simulink model "xieboduoji_13fangzhennow"  (R2023a)
settings: Solver=ode4  StartTime=0.0  StopTime=2.2  FixedStep=5e-7  RelTol=1e-3
undefined symbols (not defined in the file or in its folder): magnitude
libraries: simulink x417, spsRMSLib x70, spsCurrentMeasurementLib x32, spsVoltageMeasurementLib x31, powerlib_meascontrol x24, spsFourierLib x21, spsGroundLib x19, spsThreePhasePISectionLineLib x17, spsThreePhaseSeriesRLCBranchLib x14, spsdq0toAlphaBetaZeroLib x13, spsSeriesRLCBranchLib x11, spsUniversalBridgeLib x11
(part 10 of 12)

== system xieboduoji_13fangzhennow/node3/PV15kW2/谐波检测/DFT6-24A2/Sub5 ==
  In1 : Inport
  Constant{10,12,15,17} (4 alike) : Constant  Value=100*pi
  Constant11 : Constant  Value=19
  Cos : Trigonometry  Operator=cos
  Cos1 : Trigonometry  Operator=cos
  Cos2 : Trigonometry
  Cos3 : Trigonometry
  Delay : Delay  DelayLength=400  SampleTime=5e-5
  Delay1 : Delay  DelayLength=1  SampleTime=5e-5
  Delay2 : Delay  DelayLength=1  SampleTime=5e-5
  Divide{,1..3} (4 alike) : Product  Inputs=***
  Dot Product{,1..2,4} (4 alike) : DotProduct  OutDataTypeStr=Inherit: Inherit via internal rule
  Gain : Gain  Gain=2/400
  Gain10 : Gain  Gain=2/400
  Ramp{,1..3} (4 alike) : simulink/Sources/Ramp  slope=1  start=0  InitialOutput=0
  Sum18 : Sum  Inputs=|++
  Sum2 : Sum  Inputs=-+|
  Sum3 : Sum  Inputs=|++
  Sum9 : Sum  Inputs=|++
  Out1 : Outport
  wires:
  [thk] -> Divide/1
  Constant11/1 -> [thk]
  Sum9/1 -> Out1/1
  Dot Product1/1 -> Sum9/1
  Gain/1 -> Sum3/1
  Ramp2/1 -> Divide2/3
  Constant10/1 -> Divide/2
  Delay2/1 -> Sum18/2
  Gain10/1 -> Sum18/1
  Sum3/1 -> Delay1/1, Dot Product1/2
  Delay/1 -> Sum2/1
  Divide1/1 -> Cos1/1
  Ramp1/1 -> Divide1/3
  Constant12/1 -> Divide1/2
  Divide2/1 -> Cos2/1
  Cos3/1 -> Dot Product4/2
  Dot Product2/1 -> Gain10/1
  Cos2/1 -> Dot Product2/2
  Delay1/1 -> Sum3/2
  Divide3/1 -> Cos3/1
  Ramp3/1 -> Divide3/3
  [thk] -> Divide1/1
  Dot Product4/1 -> Sum9/2
  [thk] -> Divide2/1
  [thk] -> Divide3/1
  Sum18/1 -> Delay2/1, Dot Product4/1
  Constant15/1 -> Divide2/2
  In1/1 -> Sum2/2, Delay/1
  Cos1/1 -> Dot Product1/1
  Dot Product/1 -> Gain/1
  Cos/1 -> Dot Product/1
  Divide/1 -> Cos/1
  Sum2/1 -> Dot Product/2, Dot Product2/1
  Ramp/1 -> Divide/3
  Constant17/1 -> Divide3/2

== system xieboduoji_13fangzhennow/node3/PV15kW2/谐波检测/DFT6-24A3/Sub ==
  In1 : Inport
  Constant{10,12,15,17} (4 alike) : Constant  Value=100*pi
  Constant11 : Constant  Value=5
  Cos : Trigonometry  Operator=cos
  Cos1 : Trigonometry  Operator=cos
  Cos2 : Trigonometry
  Cos3 : Trigonometry
  Delay : Delay  DelayLength=400  SampleTime=5e-5
  Delay1 : Delay  DelayLength=1  SampleTime=5e-5
  Delay2 : Delay  DelayLength=1  SampleTime=5e-5
  Divide{,1..3} (4 alike) : Product  Inputs=***
  Dot Product{,1..2,4} (4 alike) : DotProduct  OutDataTypeStr=Inherit: Inherit via internal rule
  Gain : Gain  Gain=2/400
  Gain10 : Gain  Gain=2/400
  Ramp{,1..3} (4 alike) : simulink/Sources/Ramp  slope=1  start=0  InitialOutput=0
  Sum18 : Sum  Inputs=|++
  Sum2 : Sum  Inputs=-+|
  Sum3 : Sum  Inputs=|++
  Sum9 : Sum  Inputs=|++
  Out1 : Outport
  wires:
  Constant17/1 -> Divide3/2
  Ramp/1 -> Divide/3
  Sum2/1 -> Dot Product2/1, Dot Product/2
  Divide/1 -> Cos/1
  Cos/1 -> Dot Product/1
  Dot Product/1 -> Gain/1
  Cos1/1 -> Dot Product1/1
  In1/1 -> Delay/1, Sum2/2
  Constant15/1 -> Divide2/2
  Sum18/1 -> Dot Product4/1, Delay2/1
  [thk] -> Divide3/1
  [thk] -> Divide2/1
  Dot Product4/1 -> Sum9/2
  [thk] -> Divide1/1
  Ramp3/1 -> Divide3/3
  Divide3/1 -> Cos3/1
  Delay1/1 -> Sum3/2
  Cos2/1 -> Dot Product2/2
  Dot Product2/1 -> Gain10/1
  Cos3/1 -> Dot Product4/2
  Divide2/1 -> Cos2/1
  Constant12/1 -> Divide1/2
  Ramp1/1 -> Divide1/3
  Divide1/1 -> Cos1/1
  Delay/1 -> Sum2/1
  Sum3/1 -> Dot Product1/2, Delay1/1
  Gain10/1 -> Sum18/1
  Delay2/1 -> Sum18/2
  Constant10/1 -> Divide/2
  Ramp2/1 -> Divide2/3
  Gain/1 -> Sum3/1
  Dot Product1/1 -> Sum9/1
  Sum9/1 -> Out1/1
  Constant11/1 -> [thk]
  [thk] -> Divide/1

== system xieboduoji_13fangzhennow/node3/PV15kW2/谐波检测/DFT6-24A3/Sub1 ==
  In1 : Inport
  Constant{10,12,15,17} (4 alike) : Constant  Value=100*pi
  Constant11 : Constant  Value=7
  Cos : Trigonometry  Operator=cos
  Cos1 : Trigonometry  Operator=cos
  Cos2 : Trigonometry
  Cos3 : Trigonometry
  Delay : Delay  DelayLength=400  SampleTime=5e-5
  Delay1 : Delay  DelayLength=1  SampleTime=5e-5
  Delay2 : Delay  DelayLength=1  SampleTime=5e-5
  Divide{,1..3} (4 alike) : Product  Inputs=***
  Dot Product{,1..2,4} (4 alike) : DotProduct  OutDataTypeStr=Inherit: Inherit via internal rule
  Gain : Gain  Gain=2/400
  Gain10 : Gain  Gain=2/400
  Ramp{,1..3} (4 alike) : simulink/Sources/Ramp  slope=1  start=0  InitialOutput=0
  Sum18 : Sum  Inputs=|++
  Sum2 : Sum  Inputs=-+|
  Sum3 : Sum  Inputs=|++
  Sum9 : Sum  Inputs=|++
  Out1 : Outport
  wires:
  [thk] -> Divide/1
  Constant11/1 -> [thk]
  Sum9/1 -> Out1/1
  Dot Product1/1 -> Sum9/1
  Gain/1 -> Sum3/1
  Ramp2/1 -> Divide2/3
  Constant10/1 -> Divide/2
  Delay2/1 -> Sum18/2
  Gain10/1 -> Sum18/1
  Sum3/1 -> Delay1/1, Dot Product1/2
  Delay/1 -> Sum2/1
  Divide1/1 -> Cos1/1
  Ramp1/1 -> Divide1/3
  Constant12/1 -> Divide1/2
  Divide2/1 -> Cos2/1
  Cos3/1 -> Dot Product4/2
  Dot Product2/1 -> Gain10/1
  Cos2/1 -> Dot Product2/2
  Delay1/1 -> Sum3/2
  Divide3/1 -> Cos3/1
  Ramp3/1 -> Divide3/3
  [thk] -> Divide1/1
  Dot Product4/1 -> Sum9/2
  [thk] -> Divide2/1
  [thk] -> Divide3/1
  Sum18/1 -> Delay2/1, Dot Product4/1
  Constant15/1 -> Divide2/2
  In1/1 -> Sum2/2, Delay/1
  Cos1/1 -> Dot Product1/1
  Dot Product/1 -> Gain/1
  Cos/1 -> Dot Product/1
  Divide/1 -> Cos/1
  Sum2/1 -> Dot Product/2, Dot Product2/1
  Ramp/1 -> Divide/3
  Constant17/1 -> Divide3/2

== system xieboduoji_13fangzhennow/node3/PV15kW2/谐波检测/DFT6-24A3/Sub2 ==
  In1 : Inport
  Constant{10,12,15,17} (4 alike) : Constant  Value=100*pi
  Constant11 : Constant  Value=11
  Cos : Trigonometry  Operator=cos
  Cos1 : Trigonometry  Operator=cos
  Cos2 : Trigonometry
  Cos3 : Trigonometry
  Delay : Delay  DelayLength=400  SampleTime=5e-5
  Delay1 : Delay  DelayLength=1  SampleTime=5e-5
  Delay2 : Delay  DelayLength=1  SampleTime=5e-5
  Divide{,1..3} (4 alike) : Product  Inputs=***
  Dot Product{,1..2,4} (4 alike) : DotProduct  OutDataTypeStr=Inherit: Inherit via internal rule
  Gain : Gain  Gain=2/400
  Gain10 : Gain  Gain=2/400
  Ramp{,1..3} (4 alike) : simulink/Sources/Ramp  slope=1  start=0  InitialOutput=0
  Sum18 : Sum  Inputs=|++
  Sum2 : Sum  Inputs=-+|
  Sum3 : Sum  Inputs=|++
  Sum9 : Sum  Inputs=|++
  Out1 : Outport
  wires:
  Constant17/1 -> Divide3/2
  Ramp/1 -> Divide/3
  Sum2/1 -> Dot Product2/1, Dot Product/2
  Divide/1 -> Cos/1
  Cos/1 -> Dot Product/1
  Dot Product/1 -> Gain/1
  Cos1/1 -> Dot Product1/1
  In1/1 -> Delay/1, Sum2/2
  Constant15/1 -> Divide2/2
  Sum18/1 -> Dot Product4/1, Delay2/1
  [thk] -> Divide3/1
  [thk] -> Divide2/1
  Dot Product4/1 -> Sum9/2
  [thk] -> Divide1/1
  Ramp3/1 -> Divide3/3
  Divide3/1 -> Cos3/1
  Delay1/1 -> Sum3/2
  Cos2/1 -> Dot Product2/2
  Dot Product2/1 -> Gain10/1
  Cos3/1 -> Dot Product4/2
  Divide2/1 -> Cos2/1
  Constant12/1 -> Divide1/2
  Ramp1/1 -> Divide1/3
  Divide1/1 -> Cos1/1
  Delay/1 -> Sum2/1
  Sum3/1 -> Dot Product1/2, Delay1/1
  Gain10/1 -> Sum18/1
  Delay2/1 -> Sum18/2
  Constant10/1 -> Divide/2
  Ramp2/1 -> Divide2/3
  Gain/1 -> Sum3/1
  Dot Product1/1 -> Sum9/1
  Sum9/1 -> Out1/1
  Constant11/1 -> [thk]
  [thk] -> Divide/1

== system xieboduoji_13fangzhennow/node3/PV15kW2/谐波检测/DFT6-24A3/Sub3 ==
  In1 : Inport
  Constant{10,12,15,17} (4 alike) : Constant  Value=100*pi
  Constant11 : Constant  Value=13
  Cos : Trigonometry  Operator=cos
  Cos1 : Trigonometry  Operator=cos
  Cos2 : Trigonometry
  Cos3 : Trigonometry
  Delay : Delay  DelayLength=400  SampleTime=5e-5
  Delay1 : Delay  DelayLength=1  SampleTime=5e-5
  Delay2 : Delay  DelayLength=1  SampleTime=5e-5
  Divide{,1..3} (4 alike) : Product  Inputs=***
  Dot Product{,1..2,4} (4 alike) : DotProduct  OutDataTypeStr=Inherit: Inherit via internal rule
  Gain : Gain  Gain=2/400
  Gain10 : Gain  Gain=2/400
  Ramp{,1..3} (4 alike) : simulink/Sources/Ramp  slope=1  start=0  InitialOutput=0
  Sum18 : Sum  Inputs=|++
  Sum2 : Sum  Inputs=-+|
  Sum3 : Sum  Inputs=|++
  Sum9 : Sum  Inputs=|++
  Out1 : Outport
  wires:
  [thk] -> Divide/1
  Constant11/1 -> [thk]
  Sum9/1 -> Out1/1
  Dot Product1/1 -> Sum9/1
  Gain/1 -> Sum3/1
  Ramp2/1 -> Divide2/3
  Constant10/1 -> Divide/2
  Delay2/1 -> Sum18/2
  Gain10/1 -> Sum18/1
  Sum3/1 -> Delay1/1, Dot Product1/2
  Delay/1 -> Sum2/1
  Divide1/1 -> Cos1/1
  Ramp1/1 -> Divide1/3
  Constant12/1 -> Divide1/2
  Divide2/1 -> Cos2/1
  Cos3/1 -> Dot Product4/2
  Dot Product2/1 -> Gain10/1
  Cos2/1 -> Dot Product2/2
  Delay1/1 -> Sum3/2
  Divide3/1 -> Cos3/1
  Ramp3/1 -> Divide3/3
  [thk] -> Divide1/1
  Dot Product4/1 -> Sum9/2
  [thk] -> Divide2/1
  [thk] -> Divide3/1
  Sum18/1 -> Delay2/1, Dot Product4/1
  Constant15/1 -> Divide2/2
  In1/1 -> Sum2/2, Delay/1
  Cos1/1 -> Dot Product1/1
  Dot Product/1 -> Gain/1
  Cos/1 -> Dot Product/1
  Divide/1 -> Cos/1
  Sum2/1 -> Dot Product/2, Dot Product2/1
  Ramp/1 -> Divide/3
  Constant17/1 -> Divide3/2

== system xieboduoji_13fangzhennow/node3/PV15kW2/谐波检测/DFT6-24A3/Sub4 ==
  In1 : Inport
  Constant{10,12,15,17} (4 alike) : Constant  Value=100*pi
  Constant11 : Constant  Value=17
  Cos : Trigonometry  Operator=cos
  Cos1 : Trigonometry  Operator=cos
  Cos2 : Trigonometry
  Cos3 : Trigonometry
  Delay : Delay  DelayLength=400  SampleTime=5e-5
  Delay1 : Delay  DelayLength=1  SampleTime=5e-5
  Delay2 : Delay  DelayLength=1  SampleTime=5e-5
  Divide{,1..3} (4 alike) : Product  Inputs=***
  Dot Product{,1..2,4} (4 alike) : DotProduct  OutDataTypeStr=Inherit: Inherit via internal rule
  Gain : Gain  Gain=2/400
  Gain10 : Gain  Gain=2/400
  Ramp{,1..3} (4 alike) : simulink/Sources/Ramp  slope=1  start=0  InitialOutput=0
  Sum18 : Sum  Inputs=|++
  Sum2 : Sum  Inputs=-+|
  Sum3 : Sum  Inputs=|++
  Sum9 : Sum  Inputs=|++
  Out1 : Outport
  wires:
  Constant17/1 -> Divide3/2
  Ramp/1 -> Divide/3
  Sum2/1 -> Dot Product2/1, Dot Product/2
  Divide/1 -> Cos/1
  Cos/1 -> Dot Product/1
  Dot Product/1 -> Gain/1
  Cos1/1 -> Dot Product1/1
  In1/1 -> Delay/1, Sum2/2
  Constant15/1 -> Divide2/2
  Sum18/1 -> Dot Product4/1, Delay2/1
  [thk] -> Divide3/1
  [thk] -> Divide2/1
  Dot Product4/1 -> Sum9/2
  [thk] -> Divide1/1
  Ramp3/1 -> Divide3/3
  Divide3/1 -> Cos3/1
  Delay1/1 -> Sum3/2
  Cos2/1 -> Dot Product2/2
  Dot Product2/1 -> Gain10/1
  Cos3/1 -> Dot Product4/2
  Divide2/1 -> Cos2/1
  Constant12/1 -> Divide1/2
  Ramp1/1 -> Divide1/3
  Divide1/1 -> Cos1/1
  Delay/1 -> Sum2/1
  Sum3/1 -> Dot Product1/2, Delay1/1
  Gain10/1 -> Sum18/1
  Delay2/1 -> Sum18/2
  Constant10/1 -> Divide/2
  Ramp2/1 -> Divide2/3
  Gain/1 -> Sum3/1
  Dot Product1/1 -> Sum9/1
  Sum9/1 -> Out1/1
  Constant11/1 -> [thk]
  [thk] -> Divide/1

== system xieboduoji_13fangzhennow/node3/PV15kW2/谐波检测/DFT6-24A3/Sub5 ==
  In1 : Inport
  Constant{10,12,15,17} (4 alike) : Constant  Value=100*pi
  Constant11 : Constant  Value=19
  Cos : Trigonometry  Operator=cos
  Cos1 : Trigonometry  Operator=cos
  Cos2 : Trigonometry
  Cos3 : Trigonometry
  Delay : Delay  DelayLength=400  SampleTime=5e-5
  Delay1 : Delay  DelayLength=1  SampleTime=5e-5
  Delay2 : Delay  DelayLength=1  SampleTime=5e-5
  Divide{,1..3} (4 alike) : Product  Inputs=***
  Dot Product{,1..2,4} (4 alike) : DotProduct  OutDataTypeStr=Inherit: Inherit via internal rule
  Gain : Gain  Gain=2/400
  Gain10 : Gain  Gain=2/400
  Ramp{,1..3} (4 alike) : simulink/Sources/Ramp  slope=1  start=0  InitialOutput=0
  Sum18 : Sum  Inputs=|++
  Sum2 : Sum  Inputs=-+|
  Sum3 : Sum  Inputs=|++
  Sum9 : Sum  Inputs=|++
  Out1 : Outport
  wires:
  [thk] -> Divide/1
  Constant11/1 -> [thk]
  Sum9/1 -> Out1/1
  Dot Product1/1 -> Sum9/1
  Gain/1 -> Sum3/1
  Ramp2/1 -> Divide2/3
  Constant10/1 -> Divide/2
  Delay2/1 -> Sum18/2
  Gain10/1 -> Sum18/1
  Sum3/1 -> Delay1/1, Dot Product1/2
  Delay/1 -> Sum2/1
  Divide1/1 -> Cos1/1
  Ramp1/1 -> Divide1/3
  Constant12/1 -> Divide1/2
  Divide2/1 -> Cos2/1
  Cos3/1 -> Dot Product4/2
  Dot Product2/1 -> Gain10/1
  Cos2/1 -> Dot Product2/2
  Delay1/1 -> Sum3/2
  Divide3/1 -> Cos3/1
  Ramp3/1 -> Divide3/3
  [thk] -> Divide1/1
  Dot Product4/1 -> Sum9/2
  [thk] -> Divide2/1
  [thk] -> Divide3/1
  Sum18/1 -> Delay2/1, Dot Product4/1
  Constant15/1 -> Divide2/2
  In1/1 -> Sum2/2, Delay/1
  Cos1/1 -> Dot Product1/1
  Dot Product/1 -> Gain/1
  Cos/1 -> Dot Product/1
  Divide/1 -> Cos/1
  Sum2/1 -> Dot Product/2, Dot Product2/1
  Ramp/1 -> Divide/3
  Constant17/1 -> Divide3/2

== system xieboduoji_13fangzhennow/node3/PV15kW2/谐波检测/DFT6-24A4/Sub ==
  In1 : Inport
  Constant{10,12,15,17} (4 alike) : Constant  Value=100*pi
  Constant11 : Constant  Value=5
  Cos : Trigonometry  Operator=cos
  Cos1 : Trigonometry  Operator=cos
  Cos2 : Trigonometry
  Cos3 : Trigonometry
  Delay : Delay  DelayLength=400  SampleTime=5e-5
  Delay1 : Delay  DelayLength=1  SampleTime=5e-5
  Delay2 : Delay  DelayLength=1  SampleTime=5e-5
  Divide{,1..3} (4 alike) : Product  Inputs=***
  Dot Product{,1..2,4} (4 alike) : DotProduct  OutDataTypeStr=Inherit: Inherit via internal rule
  Gain : Gain  Gain=2/400
  Gain10 : Gain  Gain=2/400
  Ramp{,1..3} (4 alike) : simulink/Sources/Ramp  slope=1  start=0  InitialOutput=0
  Sum18 : Sum  Inputs=|++
  Sum2 : Sum  Inputs=-+|
  Sum3 : Sum  Inputs=|++
  Sum9 : Sum  Inputs=|++
  Out1 : Outport
  wires:
  [thk] -> Divide/1
  Constant11/1 -> [thk]
  Sum9/1 -> Out1/1
  Dot Product1/1 -> Sum9/1
  Gain/1 -> Sum3/1
  Ramp2/1 -> Divide2/3
  Constant10/1 -> Divide/2
  Delay2/1 -> Sum18/2
  Gain10/1 -> Sum18/1
  Sum3/1 -> Delay1/1, Dot Product1/2
  Delay/1 -> Sum2/1
  Divide1/1 -> Cos1/1
  Ramp1/1 -> Divide1/3
  Constant12/1 -> Divide1/2
  Divide2/1 -> Cos2/1
  Cos3/1 -> Dot Product4/2
  Dot Product2/1 -> Gain10/1
  Cos2/1 -> Dot Product2/2
  Delay1/1 -> Sum3/2
  Divide3/1 -> Cos3/1
  Ramp3/1 -> Divide3/3
  [thk] -> Divide1/1
  Dot Product4/1 -> Sum9/2
  [thk] -> Divide2/1
  [thk] -> Divide3/1
  Sum18/1 -> Delay2/1, Dot Product4/1
  Constant15/1 -> Divide2/2
  In1/1 -> Sum2/2, Delay/1
  Cos1/1 -> Dot Product1/1
  Dot Product/1 -> Gain/1
  Cos/1 -> Dot Product/1
  Divide/1 -> Cos/1
  Sum2/1 -> Dot Product/2, Dot Product2/1
  Ramp/1 -> Divide/3
  Constant17/1 -> Divide3/2

== system xieboduoji_13fangzhennow/node3/PV15kW2/谐波检测/DFT6-24A4/Sub1 ==
  In1 : Inport
  Constant{10,12,15,17} (4 alike) : Constant  Value=100*pi
  Constant11 : Constant  Value=7
  Cos : Trigonometry  Operator=cos
  Cos1 : Trigonometry  Operator=cos
  Cos2 : Trigonometry
  Cos3 : Trigonometry
  Delay : Delay  DelayLength=400  SampleTime=5e-5
  Delay1 : Delay  DelayLength=1  SampleTime=5e-5
  Delay2 : Delay  DelayLength=1  SampleTime=5e-5
  Divide{,1..3} (4 alike) : Product  Inputs=***
  Dot Product{,1..2,4} (4 alike) : DotProduct  OutDataTypeStr=Inherit: Inherit via internal rule
  Gain : Gain  Gain=2/400
  Gain10 : Gain  Gain=2/400
  Ramp{,1..3} (4 alike) : simulink/Sources/Ramp  slope=1  start=0  InitialOutput=0
  Sum18 : Sum  Inputs=|++
  Sum2 : Sum  Inputs=-+|
  Sum3 : Sum  Inputs=|++
  Sum9 : Sum  Inputs=|++
  Out1 : Outport
  wires:
  Constant17/1 -> Divide3/2
  Ramp/1 -> Divide/3
  Sum2/1 -> Dot Product2/1, Dot Product/2
  Divide/1 -> Cos/1
  Cos/1 -> Dot Product/1
  Dot Product/1 -> Gain/1
  Cos1/1 -> Dot Product1/1
  In1/1 -> Delay/1, Sum2/2
  Constant15/1 -> Divide2/2
  Sum18/1 -> Dot Product4/1, Delay2/1
  [thk] -> Divide3/1
  [thk] -> Divide2/1
  Dot Product4/1 -> Sum9/2
  [thk] -> Divide1/1
  Ramp3/1 -> Divide3/3
  Divide3/1 -> Cos3/1
  Delay1/1 -> Sum3/2
  Cos2/1 -> Dot Product2/2
  Dot Product2/1 -> Gain10/1
  Cos3/1 -> Dot Product4/2
  Divide2/1 -> Cos2/1
  Constant12/1 -> Divide1/2
  Ramp1/1 -> Divide1/3
  Divide1/1 -> Cos1/1
  Delay/1 -> Sum2/1
  Sum3/1 -> Dot Product1/2, Delay1/1
  Gain10/1 -> Sum18/1
  Delay2/1 -> Sum18/2
  Constant10/1 -> Divide/2
  Ramp2/1 -> Divide2/3
  Gain/1 -> Sum3/1
  Dot Product1/1 -> Sum9/1
  Sum9/1 -> Out1/1
  Constant11/1 -> [thk]
  [thk] -> Divide/1

== system xieboduoji_13fangzhennow/node3/PV15kW2/谐波检测/DFT6-24A4/Sub2 ==
  In1 : Inport
  Constant{10,12,15,17} (4 alike) : Constant  Value=100*pi
  Constant11 : Constant  Value=11
  Cos : Trigonometry  Operator=cos
  Cos1 : Trigonometry  Operator=cos
  Cos2 : Trigonometry
  Cos3 : Trigonometry
  Delay : Delay  DelayLength=400  SampleTime=5e-5
  Delay1 : Delay  DelayLength=1  SampleTime=5e-5
  Delay2 : Delay  DelayLength=1  SampleTime=5e-5
  Divide{,1..3} (4 alike) : Product  Inputs=***
  Dot Product{,1..2,4} (4 alike) : DotProduct  OutDataTypeStr=Inherit: Inherit via internal rule
  Gain : Gain  Gain=2/400
  Gain10 : Gain  Gain=2/400
  Ramp{,1..3} (4 alike) : simulink/Sources/Ramp  slope=1  start=0  InitialOutput=0
  Sum18 : Sum  Inputs=|++
  Sum2 : Sum  Inputs=-+|
  Sum3 : Sum  Inputs=|++
  Sum9 : Sum  Inputs=|++
  Out1 : Outport
  wires:
  [thk] -> Divide/1
  Constant11/1 -> [thk]
  Sum9/1 -> Out1/1
  Dot Product1/1 -> Sum9/1
  Gain/1 -> Sum3/1
  Ramp2/1 -> Divide2/3
  Constant10/1 -> Divide/2
  Delay2/1 -> Sum18/2
  Gain10/1 -> Sum18/1
  Sum3/1 -> Delay1/1, Dot Product1/2
  Delay/1 -> Sum2/1
  Divide1/1 -> Cos1/1
  Ramp1/1 -> Divide1/3
  Constant12/1 -> Divide1/2
  Divide2/1 -> Cos2/1
  Cos3/1 -> Dot Product4/2
  Dot Product2/1 -> Gain10/1
  Cos2/1 -> Dot Product2/2
  Delay1/1 -> Sum3/2
  Divide3/1 -> Cos3/1
  Ramp3/1 -> Divide3/3
  [thk] -> Divide1/1
  Dot Product4/1 -> Sum9/2
  [thk] -> Divide2/1
  [thk] -> Divide3/1
  Sum18/1 -> Delay2/1, Dot Product4/1
  Constant15/1 -> Divide2/2
  In1/1 -> Sum2/2, Delay/1
  Cos1/1 -> Dot Product1/1
  Dot Product/1 -> Gain/1
  Cos/1 -> Dot Product/1
  Divide/1 -> Cos/1
  Sum2/1 -> Dot Product/2, Dot Product2/1
  Ramp/1 -> Divide/3
  Constant17/1 -> Divide3/2

== system xieboduoji_13fangzhennow/node3/PV15kW2/谐波检测/DFT6-24A4/Sub3 ==
  In1 : Inport
  Constant{10,12,15,17} (4 alike) : Constant  Value=100*pi
  Constant11 : Constant  Value=13
  Cos : Trigonometry  Operator=cos
  Cos1 : Trigonometry  Operator=cos
  Cos2 : Trigonometry
  Cos3 : Trigonometry
  Delay : Delay  DelayLength=400  SampleTime=5e-5
  Delay1 : Delay  DelayLength=1  SampleTime=5e-5
  Delay2 : Delay  DelayLength=1  SampleTime=5e-5
  Divide{,1..3} (4 alike) : Product  Inputs=***
  Dot Product{,1..2,4} (4 alike) : DotProduct  OutDataTypeStr=Inherit: Inherit via internal rule
  Gain : Gain  Gain=2/400
  Gain10 : Gain  Gain=2/400
  Ramp{,1..3} (4 alike) : simulink/Sources/Ramp  slope=1  start=0  InitialOutput=0
  Sum18 : Sum  Inputs=|++
  Sum2 : Sum  Inputs=-+|
  Sum3 : Sum  Inputs=|++
  Sum9 : Sum  Inputs=|++
  Out1 : Outport
  wires:
  Constant17/1 -> Divide3/2
  Ramp/1 -> Divide/3
  Sum2/1 -> Dot Product2/1, Dot Product/2
  Divide/1 -> Cos/1
  Cos/1 -> Dot Product/1
  Dot Product/1 -> Gain/1
  Cos1/1 -> Dot Product1/1
  In1/1 -> Delay/1, Sum2/2
  Constant15/1 -> Divide2/2
  Sum18/1 -> Dot Product4/1, Delay2/1
  [thk] -> Divide3/1
  [thk] -> Divide2/1
  Dot Product4/1 -> Sum9/2
  [thk] -> Divide1/1
  Ramp3/1 -> Divide3/3
  Divide3/1 -> Cos3/1
  Delay1/1 -> Sum3/2
  Cos2/1 -> Dot Product2/2
  Dot Product2/1 -> Gain10/1
  Cos3/1 -> Dot Product4/2
  Divide2/1 -> Cos2/1
  Constant12/1 -> Divide1/2
  Ramp1/1 -> Divide1/3
  Divide1/1 -> Cos1/1
  Delay/1 -> Sum2/1
  Sum3/1 -> Dot Product1/2, Delay1/1
  Gain10/1 -> Sum18/1
  Delay2/1 -> Sum18/2
  Constant10/1 -> Divide/2
  Ramp2/1 -> Divide2/3
  Gain/1 -> Sum3/1
  Dot Product1/1 -> Sum9/1
  Sum9/1 -> Out1/1
  Constant11/1 -> [thk]
  [thk] -> Divide/1

== system xieboduoji_13fangzhennow/node3/PV15kW2/谐波检测/DFT6-24A4/Sub4 ==
  In1 : Inport
  Constant{10,12,15,17} (4 alike) : Constant  Value=100*pi
  Constant11 : Constant  Value=17
  Cos : Trigonometry  Operator=cos
  Cos1 : Trigonometry  Operator=cos
  Cos2 : Trigonometry
  Cos3 : Trigonometry
  Delay : Delay  DelayLength=400  SampleTime=5e-5
  Delay1 : Delay  DelayLength=1  SampleTime=5e-5
  Delay2 : Delay  DelayLength=1  SampleTime=5e-5
  Divide{,1..3} (4 alike) : Product  Inputs=***
  Dot Product{,1..2,4} (4 alike) : DotProduct  OutDataTypeStr=Inherit: Inherit via internal rule
  Gain : Gain  Gain=2/400
  Gain10 : Gain  Gain=2/400
  Ramp{,1..3} (4 alike) : simulink/Sources/Ramp  slope=1  start=0  InitialOutput=0
  Sum18 : Sum  Inputs=|++
  Sum2 : Sum  Inputs=-+|
  Sum3 : Sum  Inputs=|++
  Sum9 : Sum  Inputs=|++
  Out1 : Outport
  wires:
  [thk] -> Divide/1
  Constant11/1 -> [thk]
  Sum9/1 -> Out1/1
  Dot Product1/1 -> Sum9/1
  Gain/1 -> Sum3/1
  Ramp2/1 -> Divide2/3
  Constant10/1 -> Divide/2
  Delay2/1 -> Sum18/2
  Gain10/1 -> Sum18/1
  Sum3/1 -> Delay1/1, Dot Product1/2
  Delay/1 -> Sum2/1
  Divide1/1 -> Cos1/1
  Ramp1/1 -> Divide1/3
  Constant12/1 -> Divide1/2
  Divide2/1 -> Cos2/1
  Cos3/1 -> Dot Product4/2
  Dot Product2/1 -> Gain10/1
  Cos2/1 -> Dot Product2/2
  Delay1/1 -> Sum3/2
  Divide3/1 -> Cos3/1
  Ramp3/1 -> Divide3/3
  [thk] -> Divide1/1
  Dot Product4/1 -> Sum9/2
  [thk] -> Divide2/1
  [thk] -> Divide3/1
  Sum18/1 -> Delay2/1, Dot Product4/1
  Constant15/1 -> Divide2/2
  In1/1 -> Sum2/2, Delay/1
  Cos1/1 -> Dot Product1/1
  Dot Product/1 -> Gain/1
  Cos/1 -> Dot Product/1
  Divide/1 -> Cos/1
  Sum2/1 -> Dot Product/2, Dot Product2/1
  Ramp/1 -> Divide/3
  Constant17/1 -> Divide3/2

== system xieboduoji_13fangzhennow/node3/PV15kW2/谐波检测/DFT6-24A4/Sub5 ==
  In1 : Inport
  Constant{10,12,15,17} (4 alike) : Constant  Value=100*pi
  Constant11 : Constant  Value=19
  Cos : Trigonometry  Operator=cos
  Cos1 : Trigonometry  Operator=cos
  Cos2 : Trigonometry
  Cos3 : Trigonometry
  Delay : Delay  DelayLength=400  SampleTime=5e-5
  Delay1 : Delay  DelayLength=1  SampleTime=5e-5
  Delay2 : Delay  DelayLength=1  SampleTime=5e-5
  Divide{,1..3} (4 alike) : Product  Inputs=***
  Dot Product{,1..2,4} (4 alike) : DotProduct  OutDataTypeStr=Inherit: Inherit via internal rule
  Gain : Gain  Gain=2/400
  Gain10 : Gain  Gain=2/400
  Ramp{,1..3} (4 alike) : simulink/Sources/Ramp  slope=1  start=0  InitialOutput=0
  Sum18 : Sum  Inputs=|++
  Sum2 : Sum  Inputs=-+|
  Sum3 : Sum  Inputs=|++
  Sum9 : Sum  Inputs=|++
  Out1 : Outport
  wires:
  Constant17/1 -> Divide3/2
  Ramp/1 -> Divide/3
  Sum2/1 -> Dot Product2/1, Dot Product/2
  Divide/1 -> Cos/1
  Cos/1 -> Dot Product/1
  Dot Product/1 -> Gain/1
  Cos1/1 -> Dot Product1/1
  In1/1 -> Delay/1, Sum2/2
  Constant15/1 -> Divide2/2
  Sum18/1 -> Dot Product4/1, Delay2/1
  [thk] -> Divide3/1
  [thk] -> Divide2/1
  Dot Product4/1 -> Sum9/2
  [thk] -> Divide1/1
  Ramp3/1 -> Divide3/3
  Divide3/1 -> Cos3/1
  Delay1/1 -> Sum3/2
  Cos2/1 -> Dot Product2/2
  Dot Product2/1 -> Gain10/1
  Cos3/1 -> Dot Product4/2
  Divide2/1 -> Cos2/1
  Constant12/1 -> Divide1/2
  Ramp1/1 -> Divide1/3
  Divide1/1 -> Cos1/1
  Delay/1 -> Sum2/1
  Sum3/1 -> Dot Product1/2, Delay1/1
  Gain10/1 -> Sum18/1
  Delay2/1 -> Sum18/2
  Constant10/1 -> Divide/2
  Ramp2/1 -> Divide2/3
  Gain/1 -> Sum3/1
  Dot Product1/1 -> Sum9/1
  Sum9/1 -> Out1/1
  Constant11/1 -> [thk]
  [thk] -> Divide/1

== system xieboduoji_13fangzhennow/node3/PV15kW2/谐波检测/DFT6-24A5/Sub ==
  In1 : Inport
  Constant{1..3,10} (4 alike) : Constant  Value=2*100*pi
  Constant11 : Constant  Value=3
  Cos : Trigonometry  Operator=cos
  Cos1 : Trigonometry  Operator=cos
  Cos2 : Trigonometry
  Cos3 : Trigonometry
  Delay : Delay  DelayLength=200  SampleTime=5e-5
  Delay1 : Delay  DelayLength=1  SampleTime=5e-5
  Delay2 : Delay  DelayLength=1  SampleTime=5e-5
  Divide{,1..3} (4 alike) : Product  Inputs=***
  Dot Product{,1..2,4} (4 alike) : DotProduct  OutDataTypeStr=Inherit: Inherit via internal rule
  Gain : Gain  Gain=2/200
  Gain10 : Gain  Gain=2/200
  Ramp{,1..3} (4 alike) : simulink/Sources/Ramp  slope=1  start=0  InitialOutput=0
  Sum18 : Sum  Inputs=|++
  Sum2 : Sum  Inputs=-+|
  Sum3 : Sum  Inputs=|++
  Sum9 : Sum  Inputs=|++
  Out1 : Outport
  wires:
  [thk] -> Divide/1
  Constant11/1 -> [thk]
  Sum9/1 -> Out1/1
  Dot Product1/1 -> Sum9/1
  Gain/1 -> Sum3/1
  Ramp2/1 -> Divide2/3
  Constant10/1 -> Divide/2
  Delay2/1 -> Sum18/2
  Gain10/1 -> Sum18/1
  Sum3/1 -> Delay1/1, Dot Product1/2
  Delay/1 -> Sum2/1
  Divide1/1 -> Cos1/1
  Ramp1/1 -> Divide1/3
  Constant1/1 -> Divide1/2
  Divide2/1 -> Cos2/1
  Cos3/1 -> Dot Product4/2
  Dot Product2/1 -> Gain10/1
  Cos2/1 -> Dot Product2/2
  Delay1/1 -> Sum3/2
  Divide3/1 -> Cos3/1
  Ramp3/1 -> Divide3/3
  [thk] -> Divide1/1
  Dot Product4/1 -> Sum9/2
  [thk] -> Divide2/1
  [thk] -> Divide3/1
  Sum18/1 -> Delay2/1, Dot Product4/1
  Constant3/1 -> Divide2/2
  In1/1 -> Sum2/2, Delay/1
  Cos1/1 -> Dot Product1/1
  Dot Product/1 -> Gain/1
  Cos/1 -> Dot Product/1
  Divide/1 -> Cos/1
  Sum2/1 -> Dot Product/2, Dot Product2/1
  Ramp/1 -> Divide/3
  Constant2/1 -> Divide3/2

== system xieboduoji_13fangzhennow/node3/PV15kW2/谐波检测/DFT6-24A5/Sub1 ==
  In1 : Inport
  Constant{1..3,10} (4 alike) : Constant  Value=2*100*pi
  Constant11 : Constant  Value=6
  Cos : Trigonometry  Operator=cos
  Cos1 : Trigonometry  Operator=cos
  Cos2 : Trigonometry
  Cos3 : Trigonometry
  Delay : Delay  DelayLength=200  SampleTime=5e-5
  Delay1 : Delay  DelayLength=1  SampleTime=5e-5
  Delay2 : Delay  DelayLength=1  SampleTime=5e-5
  Divide{,1..3} (4 alike) : Product  Inputs=***
  Dot Product{,1..2,4} (4 alike) : DotProduct  OutDataTypeStr=Inherit: Inherit via internal rule
  Gain : Gain  Gain=2/200
  Gain10 : Gain  Gain=2/200
  Ramp{,1..3} (4 alike) : simulink/Sources/Ramp  slope=1  start=0  InitialOutput=0
  Sum18 : Sum  Inputs=|++
  Sum2 : Sum  Inputs=-+|
  Sum3 : Sum  Inputs=|++
  Sum9 : Sum  Inputs=|++
  Out1 : Outport
  wires:
  Constant2/1 -> Divide3/2
  Ramp/1 -> Divide/3
  Sum2/1 -> Dot Product2/1, Dot Product/2
  Divide/1 -> Cos/1
  Cos/1 -> Dot Product/1
  Dot Product/1 -> Gain/1
  Cos1/1 -> Dot Product1/1
  In1/1 -> Delay/1, Sum2/2
  Constant3/1 -> Divide2/2
  Sum18/1 -> Dot Product4/1, Delay2/1
  [thk] -> Divide3/1
  [thk] -> Divide2/1
  Dot Product4/1 -> Sum9/2
  [thk] -> Divide1/1
  Ramp3/1 -> Divide3/3
  Divide3/1 -> Cos3/1
  Delay1/1 -> Sum3/2
  Cos2/1 -> Dot Product2/2
  Dot Product2/1 -> Gain10/1
  Cos3/1 -> Dot Product4/2
  Divide2/1 -> Cos2/1
  Constant1/1 -> Divide1/2
  Ramp1/1 -> Divide1/3
  Divide1/1 -> Cos1/1
  Delay/1 -> Sum2/1
  Sum3/1 -> Dot Product1/2, Delay1/1
  Gain10/1 -> Sum18/1
  Delay2/1 -> Sum18/2
  Constant10/1 -> Divide/2
  Ramp2/1 -> Divide2/3
  Gain/1 -> Sum3/1
  Dot Product1/1 -> Sum9/1
  Sum9/1 -> Out1/1
  Constant11/1 -> [thk]
  [thk] -> Divide/1

== system xieboduoji_13fangzhennow/node3/PV15kW2/谐波检测/DFT6-24A5/Sub3 ==
  In1 : Inport
  Constant{1..3,10} (4 alike) : Constant  Value=2*100*pi
  Constant11 : Constant  Value=9
  Constant4 : Constant  Commented=on  Value=pi*0.3333
  Constant5 : Constant  Commented=on  Value=pi*0.3333
  Cos : Trigonometry  Operator=cos
  Cos1 : Trigonometry  Operator=cos
  Cos2 : Trigonometry
  Cos3 : Trigonometry
  Delay : Delay  DelayLength=200  SampleTime=5e-5
  Delay1 : Delay  DelayLength=1  SampleTime=5e-5
  Delay2 : Delay  DelayLength=1  SampleTime=5e-5
  Divide{,1..3} (4 alike) : Product  Inputs=***
  Dot Product{,1..2,4} (4 alike) : DotProduct  OutDataTypeStr=Inherit: Inherit via internal rule
  Gain : Gain  Gain=2/200
  Gain10 : Gain  Gain=2/200
  Ramp{,1..3} (4 alike) : simulink/Sources/Ramp  slope=1  start=0  InitialOutput=0
  Sum{1,3..4,9,18} (5 alike) : Sum  Inputs=|++
  Sum2 : Sum  Inputs=-+|
  Out1 : Outport
  wires:
  Constant2/1 -> Divide3/2
  Ramp/1 -> Divide/3
  Sum2/1 -> Dot Product2/1, Dot Product/2
  Divide/1 -> Cos/1
  Cos/1 -> Dot Product/1
  Dot Product/1 -> Gain/1
  Cos1/1 -> Dot Product1/1
  In1/1 -> Delay/1, Sum2/2
  Constant3/1 -> Divide2/2
  Sum18/1 -> Delay2/1, Dot Product4/1
  [thk] -> Divide3/1
  [thk] -> Divide2/1
  Dot Product4/1 -> Sum9/2
  [thk] -> Divide1/1
  Ramp3/1 -> Divide3/3
  Delay1/1 -> Sum3/2
  Cos2/1 -> Dot Product2/2
  Dot Product2/1 -> Gain10/1
  Cos3/1 -> Dot Product4/2
  Divide2/1 -> Cos2/1
  Constant1/1 -> Divide1/2
  Ramp1/1 -> Divide1/3
  Delay/1 -> Sum2/1
  Sum3/1 -> Dot Product1/2, Delay1/1
  Gain10/1 -> Sum18/1
  Delay2/1 -> Sum18/2
  Constant10/1 -> Divide/2
  Ramp2/1 -> Divide2/3
  Gain/1 -> Sum3/1
  Dot Product1/1 -> Sum9/1
  Sum9/1 -> Out1/1
  Constant11/1 -> [thk]
  [thk] -> Divide/1
  Divide1/1 -> Sum1/1
  Sum1/1 -> Cos1/1
  Constant4/1 -> Sum1/2
  Divide3/1 -> Sum4/1
  Sum4/1 -> Cos3/1
  Constant5/1 -> Sum4/2

== system xieboduoji_13fangzhennow/node3/PV15kW2/谐波检测/Subsystem2/RMS1 ==
  u : Inport
  Trigger : TriggerPort  VariantControl=(inherit)
  Embedded MATLAB Function : MATLAB Function  TreatAsAtomicUnit=on
  ki : Outport  VectorParamsAs1DForOutWhenUnconnected=off
  wires:
  Embedded MATLAB Function/1(ki) -> ki/1
  u/1 -> Embedded MATLAB Function/1(u)

== system xieboduoji_13fangzhennow/node3/PV15kW2/谐波检测/Subsystem3/RMS1 ==
  u : Inport
  Trigger : TriggerPort  VariantControl=(inherit)
  Embedded MATLAB Function : MATLAB Function  TreatAsAtomicUnit=on
  y : Outport  VectorParamsAs1DForOutWhenUnconnected=off
  ki : Outport  Port=2  VectorParamsAs1DForOutWhenUnconnected=off
  wires:
  Embedded MATLAB Function/1(ki) -> ki/1
  Embedded MATLAB Function/2(y) -> y/1
  u/1 -> Embedded MATLAB Function/1(u)

== system xieboduoji_13fangzhennow/node3/PV15kW3/谐波检测/Subsystem/Sub ==
  In1 : Inport
  Constant1 : Constant  Value=-60*pi/180
  Constant{10,12,15,17} (4 alike) : Constant  Value=100*pi
  Constant11 : Constant  Value=5
  Constant2 : Constant  Value=-60*pi/180
  Cos : Trigonometry  Operator=cos
  Cos1 : Trigonometry  Operator=cos
  Cos2 : Trigonometry
  Cos3 : Trigonometry
  Delay : Delay  DelayLength=400  SampleTime=5e-5
  Delay1 : Delay  DelayLength=1  SampleTime=5e-5
  Delay2 : Delay  DelayLength=1  SampleTime=5e-5
  Divide{,1..3} (4 alike) : Product  Inputs=***
  Dot Product{,1..2,4} (4 alike) : DotProduct  OutDataTypeStr=Inherit: Inherit via internal rule
  Gain : Gain  Gain=2/400
  Gain10 : Gain  Gain=2/400
  Ramp{,1..3} (4 alike) : simulink/Sources/Ramp  slope=1  start=0  InitialOutput=0
  Sum{,1,3,9,18} (5 alike) : Sum  Inputs=|++
  Sum2 : Sum  Inputs=-+|
  u1 : Outport
  wires:
  [thk] -> Divide/1
  Constant11/1 -> [thk]
  Sum9/1 -> u1/1
  Dot Product1/1 -> Sum9/1
  Gain/1 -> Sum3/1
  Ramp2/1 -> Divide2/3
  Constant10/1 -> Divide/2
  Delay2/1 -> Sum18/2
  Gain10/1 -> Sum18/1
  Sum3/1 -> Delay1/1, Dot Product1/2
  Delay/1 -> Sum2/1
  Ramp1/1 -> Divide1/3
  Constant12/1 -> Divide1/2
  Divide2/1 -> Cos2/1
  Cos3/1 -> Dot Product4/2
  Dot Product2/1 -> Gain10/1
  Cos2/1 -> Dot Product2/2
  Delay1/1 -> Sum3/2
  Ramp3/1 -> Divide3/3
  [thk] -> Divide1/1
  Dot Product4/1 -> Sum9/2
  [thk] -> Divide2/1
  [thk] -> Divide3/1
  Sum18/1 -> Delay2/1, Dot Product4/1
  Constant15/1 -> Divide2/2
  In1/1 -> Sum2/2, Delay/1
  Dot Product/1 -> Gain/1
  Cos/1 -> Dot Product/1
  Divide/1 -> Cos/1
  Sum2/1 -> Dot Product/2, Dot Product2/1
  Ramp/1 -> Divide/3
  Constant17/1 -> Divide3/2
  Cos1/1 -> Dot Product1/1
  Divide1/1 -> Sum/1
  Sum/1 -> Cos1/1
  Sum1/1 -> Cos3/1
  Divide3/1 -> Sum1/1

== system xieboduoji_13fangzhennow/node3/PV15kW3/谐波检测/Subsystem/Sub1 ==
  In1 : Inport
  Constant1 : Constant  Value=-60*pi/180
  Constant{10,12,15,17} (4 alike) : Constant  Value=100*pi
  Constant11 : Constant  Value=7
  Constant2 : Constant  Value=-60*pi/180
  Cos : Trigonometry  Operator=cos
  Cos1 : Trigonometry  Operator=cos
  Cos2 : Trigonometry
  Cos3 : Trigonometry
  Delay : Delay  DelayLength=400  SampleTime=5e-5
  Delay1 : Delay  DelayLength=1  SampleTime=5e-5
  Delay2 : Delay  DelayLength=1  SampleTime=5e-5
  Divide{,1..3} (4 alike) : Product  Inputs=***
  Dot Product{,1..2,4} (4 alike) : DotProduct  OutDataTypeStr=Inherit: Inherit via internal rule
  Gain : Gain  Gain=2/400
  Gain10 : Gain  Gain=2/400
  Ramp{,1..3} (4 alike) : simulink/Sources/Ramp  slope=1  start=0  InitialOutput=0
  Sum{,1,3,9,18} (5 alike) : Sum  Inputs=|++
  Sum2 : Sum  Inputs=-+|
  u1 : Outport
  wires:
  Divide3/1 -> Sum1/1
  Sum1/1 -> Cos3/1
  Sum/1 -> Cos1/1
  Divide1/1 -> Sum/1
  Cos1/1 -> Dot Product1/1
  Constant17/1 -> Divide3/2
  Ramp/1 -> Divide/3
  Sum2/1 -> Dot Product2/1, Dot Product/2
  Divide/1 -> Cos/1
  Cos/1 -> Dot Product/1
  Dot Product/1 -> Gain/1
  In1/1 -> Delay/1, Sum2/2
  Constant15/1 -> Divide2/2
  Sum18/1 -> Dot Product4/1, Delay2/1
  [thk] -> Divide3/1
  [thk] -> Divide2/1
  Dot Product4/1 -> Sum9/2
  [thk] -> Divide1/1
  Ramp3/1 -> Divide3/3
  Delay1/1 -> Sum3/2
  Cos2/1 -> Dot Product2/2
  Dot Product2/1 -> Gain10/1
  Cos3/1 -> Dot Product4/2
  Divide2/1 -> Cos2/1
  Constant12/1 -> Divide1/2
  Ramp1/1 -> Divide1/3
  Delay/1 -> Sum2/1
  Sum3/1 -> Dot Product1/2, Delay1/1
  Gain10/1 -> Sum18/1
  Delay2/1 -> Sum18/2
  Constant10/1 -> Divide/2
  Ramp2/1 -> Divide2/3
  Gain/1 -> Sum3/1
  Dot Product1/1 -> Sum9/1
  Sum9/1 -> u1/1
  Constant11/1 -> [thk]
  [thk] -> Divide/1

== system xieboduoji_13fangzhennow/node3/PV15kW3/谐波检测/Subsystem/Sub10 ==
  In1 : Inport
  Constant1 : Constant  Value=10*pi/180
  Constant{10,12,15,17} (4 alike) : Constant  Value=100*pi
  Constant11 : Constant  Value=19
  Constant2 : Constant  Value=10*pi/180
  Cos : Trigonometry  Operator=cos
  Cos1 : Trigonometry  Operator=cos
  Cos2 : Trigonometry
  Cos3 : Trigonometry
  Delay : Delay  DelayLength=400  SampleTime=5e-5
  Delay1 : Delay  DelayLength=1  SampleTime=5e-5
  Delay2 : Delay  DelayLength=1  SampleTime=5e-5
  Divide{,1..3} (4 alike) : Product  Inputs=***
  Dot Product{,1..2,4} (4 alike) : DotProduct  OutDataTypeStr=Inherit: Inherit via internal rule
  Gain : Gain  Gain=2/400
  Gain10 : Gain  Gain=2/400
  Ramp{,1..3} (4 alike) : simulink/Sources/Ramp  slope=1  start=0  InitialOutput=0
  Sum{,1,3,9,18} (5 alike) : Sum  Inputs=|++
  Sum2 : Sum  Inputs=-+|
  u9 : Outport
  wires:
  [thk] -> Divide/1
  Constant11/1 -> [thk]
  Sum9/1 -> u9/1
  Dot Product1/1 -> Sum9/1
  Gain/1 -> Sum3/1
  Ramp2/1 -> Divide2/3
  Constant10/1 -> Divide/2
  Delay2/1 -> Sum18/2
  Gain10/1 -> Sum18/1
  Sum3/1 -> Delay1/1, Dot Product1/2
  Delay/1 -> Sum2/1
  Ramp1/1 -> Divide1/3
  Constant12/1 -> Divide1/2
  Divide2/1 -> Cos2/1
  Cos3/1 -> Dot Product4/2
  Dot Product2/1 -> Gain10/1
  Cos2/1 -> Dot Product2/2
  Delay1/1 -> Sum3/2
  Ramp3/1 -> Divide3/3
  [thk] -> Divide1/1
  Dot Product4/1 -> Sum9/2
  [thk] -> Divide2/1
  [thk] -> Divide3/1
  Sum18/1 -> Delay2/1, Dot Product4/1
  Constant15/1 -> Divide2/2
  In1/1 -> Sum2/2, Delay/1
  Cos1/1 -> Dot Product1/1
  Dot Product/1 -> Gain/1
  Cos/1 -> Dot Product/1
  Divide/1 -> Cos/1
  Sum2/1 -> Dot Product/2, Dot Product2/1
  Ramp/1 -> Divide/3
  Constant17/1 -> Divide3/2
  Divide1/1 -> Sum/1
  Sum/1 -> Cos1/1
  Divide3/1 -> Sum1/1
  Sum1/1 -> Cos3/1
  Constant2/1 -> Sum/2
  Constant1/1 -> Sum1/2

== system xieboduoji_13fangzhennow/node3/PV15kW3/谐波检测/Subsystem/Sub12 ==
  In1 : Inport
  Constant1 : Constant  Value=10*pi/180
  Constant{10,12,15,17} (4 alike) : Constant  Value=100*pi
  Constant11 : Constant  Value=17
  Constant2 : Constant  Value=10*pi/180
  Cos : Trigonometry  Operator=cos
  Cos1 : Trigonometry  Operator=cos
  Cos2 : Trigonometry
  Cos3 : Trigonometry
  Delay : Delay  DelayLength=400  SampleTime=5e-5
  Delay1 : Delay  DelayLength=1  SampleTime=5e-5
  Delay2 : Delay  DelayLength=1  SampleTime=5e-5
  Divide{,1..3} (4 alike) : Product  Inputs=***
  Dot Product{,1..2,4} (4 alike) : DotProduct  OutDataTypeStr=Inherit: Inherit via internal rule
  Gain : Gain  Gain=2/400
  Gain10 : Gain  Gain=2/400
  Ramp{,1..3} (4 alike) : simulink/Sources/Ramp  slope=1  start=0  InitialOutput=0
  Sum{,1,3,9,18} (5 alike) : Sum  Inputs=|++
  Sum2 : Sum  Inputs=-+|
  u9 : Outport
  wires:
  Constant1/1 -> Sum1/2
  Constant2/1 -> Sum/2
  Sum1/1 -> Cos3/1
  Divide3/1 -> Sum1/1
  Sum/1 -> Cos1/1
  Divide1/1 -> Sum/1
  Constant17/1 -> Divide3/2
  Ramp/1 -> Divide/3
  Sum2/1 -> Dot Product2/1, Dot Product/2
  Divide/1 -> Cos/1
  Cos/1 -> Dot Product/1
  Dot Product/1 -> Gain/1
  Cos1/1 -> Dot Product1/1
  In1/1 -> Delay/1, Sum2/2
  Constant15/1 -> Divide2/2
  Sum18/1 -> Dot Product4/1, Delay2/1
  [thk] -> Divide3/1
  [thk] -> Divide2/1
  Dot Product4/1 -> Sum9/2
  [thk] -> Divide1/1
  Ramp3/1 -> Divide3/3
  Delay1/1 -> Sum3/2
  Cos2/1 -> Dot Product2/2
  Dot Product2/1 -> Gain10/1
  Cos3/1 -> Dot Product4/2
  Divide2/1 -> Cos2/1
  Constant12/1 -> Divide1/2
  Ramp1/1 -> Divide1/3
  Delay/1 -> Sum2/1
  Sum3/1 -> Dot Product1/2, Delay1/1
  Gain10/1 -> Sum18/1
  Delay2/1 -> Sum18/2
  Constant10/1 -> Divide/2
  Ramp2/1 -> Divide2/3
  Gain/1 -> Sum3/1
  Dot Product1/1 -> Sum9/1
  Sum9/1 -> u9/1
  Constant11/1 -> [thk]
  [thk] -> Divide/1

== system xieboduoji_13fangzhennow/node3/PV15kW3/谐波检测/Subsystem/Sub2 ==
  In1 : Inport
  Constant1 : Constant  Value=-15*pi/180
  Constant{10,12,15,17} (4 alike) : Constant  Value=100*pi
  Constant11 : Constant  Value=11
  Constant2 : Constant  Value=-15*pi/180
  Cos : Trigonometry  Operator=cos
  Cos2 : Trigonometry
  Cos3 : Trigonometry
  Cos4 : Trigonometry  Operator=cos
  Delay : Delay  DelayLength=400  SampleTime=5e-5
  Delay1 : Delay  DelayLength=1  SampleTime=5e-5
  Delay2 : Delay  DelayLength=1  SampleTime=5e-5
  Divide{,1..3} (4 alike) : Product  Inputs=***
  Dot Product{,1..2,4} (4 alike) : DotProduct  OutDataTypeStr=Inherit: Inherit via internal rule
  Gain : Gain  Gain=2/400
  Gain10 : Gain  Gain=2/400
  Ramp{,1..3} (4 alike) : simulink/Sources/Ramp  slope=1  start=0  InitialOutput=0
  Sum{,1,3,9,18} (5 alike) : Sum  Inputs=|++
  Sum2 : Sum  Inputs=-+|
  u5 : Outport
  wires:
  [thk] -> Divide/1
  Constant11/1 -> [thk]
  Sum9/1 -> u5/1
  Dot Product1/1 -> Sum9/1
  Gain/1 -> Sum3/1
  Ramp2/1 -> Divide2/3
  Constant10/1 -> Divide/2
  Delay2/1 -> Sum18/2
  Gain10/1 -> Sum18/1
  Sum3/1 -> Delay1/1, Dot Product1/2
  Delay/1 -> Sum2/1
  Ramp1/1 -> Divide1/3
  Constant12/1 -> Divide1/2
  Divide2/1 -> Cos2/1
  Cos3/1 -> Dot Product4/2
  Dot Product2/1 -> Gain10/1
  Cos2/1 -> Dot Product2/2
  Delay1/1 -> Sum3/2
  Ramp3/1 -> Divide3/3
  [thk] -> Divide1/1
  Dot Product4/1 -> Sum9/2
  [thk] -> Divide2/1
  [thk] -> Divide3/1
  Sum18/1 -> Delay2/1, Dot Product4/1
  Constant15/1 -> Divide2/2
  In1/1 -> Sum2/2, Delay/1
  Dot Product/1 -> Gain/1
  Cos/1 -> Dot Product/1
  Divide/1 -> Cos/1
  Sum2/1 -> Dot Product/2, Dot Product2/1
  Ramp/1 -> Divide/3
  Constant17/1 -> Divide3/2
  Divide1/1 -> Sum/1
  Constant2/1 -> Sum/2
  Sum/1 -> Cos4/1
  Cos4/1 -> Dot Product1/1
  Divide3/1 -> Sum1/1
  Constant1/1 -> Sum1/2
  Sum1/1 -> Cos3/1

== system xieboduoji_13fangzhennow/node3/PV15kW3/谐波检测/Subsystem/Sub3 ==
  In1 : Inport
  Constant1 : Constant  Value=-15*pi/180
  Constant{10,12,15,17} (4 alike) : Constant  Value=100*pi
  Constant11 : Constant  Value=13
  Constant2 : Constant  Value=-15*pi/180
  Cos : Trigonometry  Operator=cos
  Cos1 : Trigonometry  Operator=cos
  Cos2 : Trigonometry
  Cos3 : Trigonometry
  Delay : Delay  DelayLength=400  SampleTime=5e-5
  Delay1 : Delay  DelayLength=1  SampleTime=5e-5
  Delay2 : Delay  DelayLength=1  SampleTime=5e-5
  Divide{,1..3} (4 alike) : Product  Inputs=***
  Dot Product{,1..2,4} (4 alike) : DotProduct  OutDataTypeStr=Inherit: Inherit via internal rule
  Gain : Gain  Gain=2/400
  Gain10 : Gain  Gain=2/400
  Ramp{,1..3} (4 alike) : simulink/Sources/Ramp  slope=1  start=0  InitialOutput=0
  Sum{,1,3,9,18} (5 alike) : Sum  Inputs=|++
  Sum2 : Sum  Inputs=-+|
  u7 : Outport
  wires:
  Constant17/1 -> Divide3/2
  Ramp/1 -> Divide/3
  Sum2/1 -> Dot Product2/1, Dot Product/2
  Divide/1 -> Cos/1
  Cos/1 -> Dot Product/1
  Dot Product/1 -> Gain/1
  Cos1/1 -> Dot Product1/1
  In1/1 -> Delay/1, Sum2/2
  Constant15/1 -> Divide2/2
  Sum18/1 -> Dot Product4/1, Delay2/1
  [thk] -> Divide3/1
  [thk] -> Divide2/1
  Dot Product4/1 -> Sum9/2
  [thk] -> Divide1/1
  Ramp3/1 -> Divide3/3
  Delay1/1 -> Sum3/2
  Cos2/1 -> Dot Product2/2
  Dot Product2/1 -> Gain10/1
  Cos3/1 -> Dot Product4/2
  Divide2/1 -> Cos2/1
  Constant12/1 -> Divide1/2
  Ramp1/1 -> Divide1/3
  Delay/1 -> Sum2/1
  Sum3/1 -> Dot Product1/2, Delay1/1
  Gain10/1 -> Sum18/1
  Delay2/1 -> Sum18/2
  Constant10/1 -> Divide/2
  Ramp2/1 -> Divide2/3
  Gain/1 -> Sum3/1
  Dot Product1/1 -> Sum9/1
  Sum9/1 -> u7/1
  Constant11/1 -> [thk]
  [thk] -> Divide/1
  Divide1/1 -> Sum/1
  Constant2/1 -> Sum/2
  Sum/1 -> Cos1/1
  Divide3/1 -> Sum1/1
  Constant1/1 -> Sum1/2
  Sum1/1 -> Cos3/1

== system xieboduoji_13fangzhennow/node3/PV15kW3/谐波检测/Subsystem/Sub4 ==
  In1 : Inport
  Constant1 : Constant  Value=10*pi/180
  Constant{10,12,15,17} (4 alike) : Constant  Value=100*pi
  Constant11 : Constant  Value=17
  Constant2 : Constant  Value=10*pi/180
  Cos : Trigonometry  Operator=cos
  Cos1 : Trigonometry  Operator=cos
  Cos2 : Trigonometry
  Cos3 : Trigonometry
  Delay : Delay  DelayLength=400  SampleTime=5e-5
  Delay1 : Delay  DelayLength=1  SampleTime=5e-5
  Delay2 : Delay  DelayLength=1  SampleTime=5e-5
  Divide{,1..3} (4 alike) : Product  Inputs=***
  Dot Product{,1..2,4} (4 alike) : DotProduct  OutDataTypeStr=Inherit: Inherit via internal rule
  Gain : Gain  Gain=2/400
  Gain10 : Gain  Gain=2/400
  Ramp{,1..3} (4 alike) : simulink/Sources/Ramp  slope=1  start=0  InitialOutput=0
  Sum{,1,3,9,18} (5 alike) : Sum  Inputs=|++
  Sum2 : Sum  Inputs=-+|
  u9 : Outport
  wires:
  [thk] -> Divide/1
  Constant11/1 -> [thk]
  Sum9/1 -> u9/1
  Dot Product1/1 -> Sum9/1
  Gain/1 -> Sum3/1
  Ramp2/1 -> Divide2/3
  Constant10/1 -> Divide/2
  Delay2/1 -> Sum18/2
  Gain10/1 -> Sum18/1
  Sum3/1 -> Delay1/1, Dot Product1/2
  Delay/1 -> Sum2/1
  Ramp1/1 -> Divide1/3
  Constant12/1 -> Divide1/2
  Divide2/1 -> Cos2/1
  Cos3/1 -> Dot Product4/2
  Dot Product2/1 -> Gain10/1
  Cos2/1 -> Dot Product2/2
  Delay1/1 -> Sum3/2
  Ramp3/1 -> Divide3/3
  [thk] -> Divide1/1
  Dot Product4/1 -> Sum9/2
  [thk] -> Divide2/1
  [thk] -> Divide3/1
  Sum18/1 -> Delay2/1, Dot Product4/1
  Constant15/1 -> Divide2/2
  In1/1 -> Sum2/2, Delay/1
  Cos1/1 -> Dot Product1/1
  Dot Product/1 -> Gain/1
  Cos/1 -> Dot Product/1
  Divide/1 -> Cos/1
  Sum2/1 -> Dot Product/2, Dot Product2/1
  Ramp/1 -> Divide/3
  Constant17/1 -> Divide3/2
  Divide1/1 -> Sum/1
  Sum/1 -> Cos1/1
  Divide3/1 -> Sum1/1
  Sum1/1 -> Cos3/1
  Constant2/1 -> Sum/2
  Constant1/1 -> Sum1/2
